simulink model "case 3"  (R2018a)
settings: Solver=VariableStepAuto  StartTime=0.0  StopTime=5  RelTol=1e-3
values from neighbouring files (symbols this model uses):
  cdcc = 0.00022    [matlab.mat]    (also in parameters.m)
  cf = 8e-05    [matlab.mat]    (also in parameters.m = 2e-05)
  iodmax = 12    [matlab.mat]    (also in parameters.m)
  iqdmax = -7.2    [matlab.mat]    (also in parameters.m)
  kiid = 0.5    [matlab.mat]    (also in parameters.m)
  kiiq = -5    [matlab.mat]    (also in parameters.m)
  kpid = 0.4    [matlab.mat]    (also in parameters.m)
  kpiq = -4    [matlab.mat]    (also in parameters.m)
  lf = 0.0075    [matlab.mat]    (also in parameters.m = 0.0015)
  ll = 1e-06    [matlab.mat]    (also in parameters.m)
  md = 0.001    [matlab.mat]    (also in parameters.m)
  nq = 0.002    [matlab.mat]    (also in parameters.m)
  p0 = 240    [matlab.mat]    (also in parameters.m)
  q0 = 60    [matlab.mat]    (also in parameters.m)
  rf = 0.0015    [matlab.mat]    (also in parameters.m)
  rl = 0.001    [matlab.mat]    (also in parameters.m)
  vdc = 200    [matlab.mat]    (also in parameters.m)
  wc = 0.000125663706144    [matlab.mat]    (also in parameters.m)
undefined symbols (not defined in the file or in its folder): DiscIntNeverNeededParam, gcbh, sps, sps_rtmsupport
libraries: powerlib_meascontrol x29, powerlib x17, simulink x6, spsVIMeasurementModel x6, spsMeanValueModel x2
(part 2 of 2)

== system case 3/Controller/Mean1/Mean1 ==
  In : Inport  SampleTime=Ts
  Model : Subsystem
  Mean : Outport  SampleTime=Ts
  wires:
  In/1 -> Model/1(In)
  Model/1(Mean) -> Mean/1

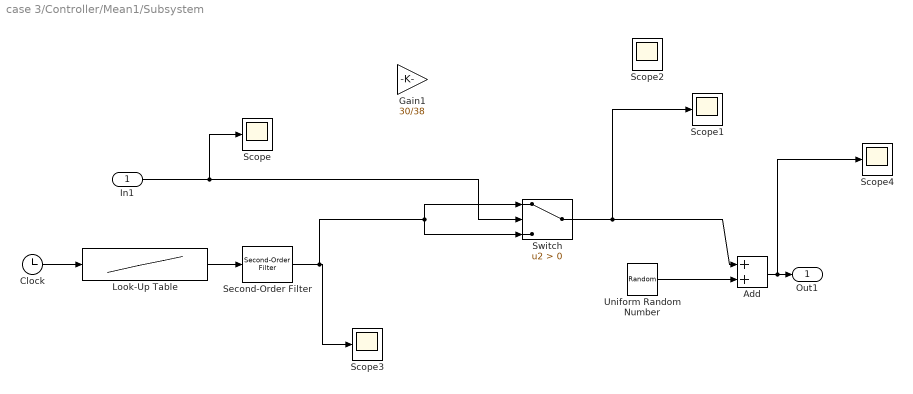
== system case 3/Controller/Mean1/Subsystem ==
  In1 : Inport
  Add : Sum
  Clock : Clock
  Gain1 : Gain  Gain=30/38
  Look-Up Table : Lookup  InputValues=[0 2 2.01 6]  Table=[-0.01 -0.01 -12 -12]  SaturateOnIntegerOverflow=on
  Scope{,1..4} (5 alike) : Scope
  Second-Order Filter : powerlib_meascontrol/Filters/Second-Order Filter  FilterType=Lowpass  Fo=10  Zeta=0.909  Ts=50e-6  Initialize=off  Vac_Init="[0,  0,  60]"  Vdc_Init=0  PlotResponse=off  FreqRange=[0, 500, 1]
      settings: SourceProductName=Simscape Power Systems  SourceProductBaseCode=PS
  Switch : Switch  Criteria=u2 > Threshold
  Uniform Random Number : UniformRandomNumber  Minimum=-0.5  Maximum=0.5  SampleTime=50e-6
  Out1 : Outport
  wires:
  Clock/1 -> Look-Up Table/1
  Look-Up Table/1 -> Second-Order Filter/1
  In1/1 -> Switch/2, Scope/1
  Second-Order Filter/1 -> Switch/1, Switch/3, Scope3/1
  Switch/1 -> Add/1, Scope1/1
  Add/1 -> Scope4/1, Out1/1
  Uniform Random Number/1 -> Add/2

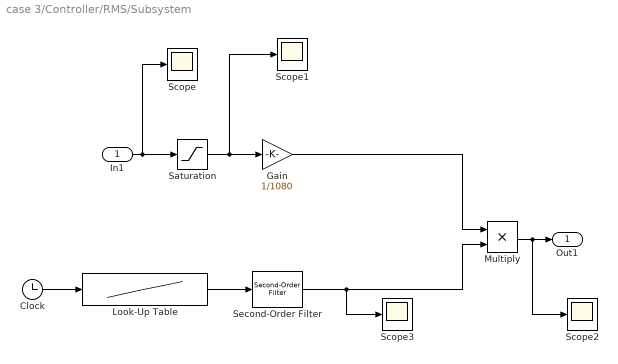
== system case 3/Controller/RMS/Subsystem ==
  In1 : Inport
  Clock : Clock
  Gain : Gain  Gain=1/1080
  Look-Up Table : Lookup  InputValues=[0 2 2.2 5]  Table=[235 235 80 120]  SaturateOnIntegerOverflow=on
  Multiply : Product
  Saturation : Saturate  UpperLimit=inf  LowerLimit=1080
  Scope{,1..3} (4 alike) : Scope
  Second-Order Filter : powerlib_meascontrol/Filters/Second-Order Filter  FilterType=Lowpass  Fo=30  Zeta=0.707  Ts=50e-6  Initialize=off  Vac_Init="[0,  0,  60]"  Vdc_Init=0  PlotResponse=off  FreqRange=[0, 500, 1]
      settings: SourceProductName=Simscape Power Systems  SourceProductBaseCode=PS
  Out1 : Outport
  wires:
  Saturation/1 -> Scope1/1, Gain/1
  In1/1 -> Scope/1, Saturation/1
  Gain/1 -> Multiply/1
  Clock/1 -> Look-Up Table/1
  Look-Up Table/1 -> Second-Order Filter/1
  Multiply/1 -> Scope2/1, Out1/1
  Second-Order Filter/1 -> Scope3/1, Multiply/2

== system case 3/Controller/RMS4/Mean1 ==
  In : Inport  SampleTime=Ts
  Model : Subsystem
  Mean : Outport  SampleTime=Ts
  wires:
  In/1 -> Model/1(In)
  Model/1(Mean) -> Mean/1

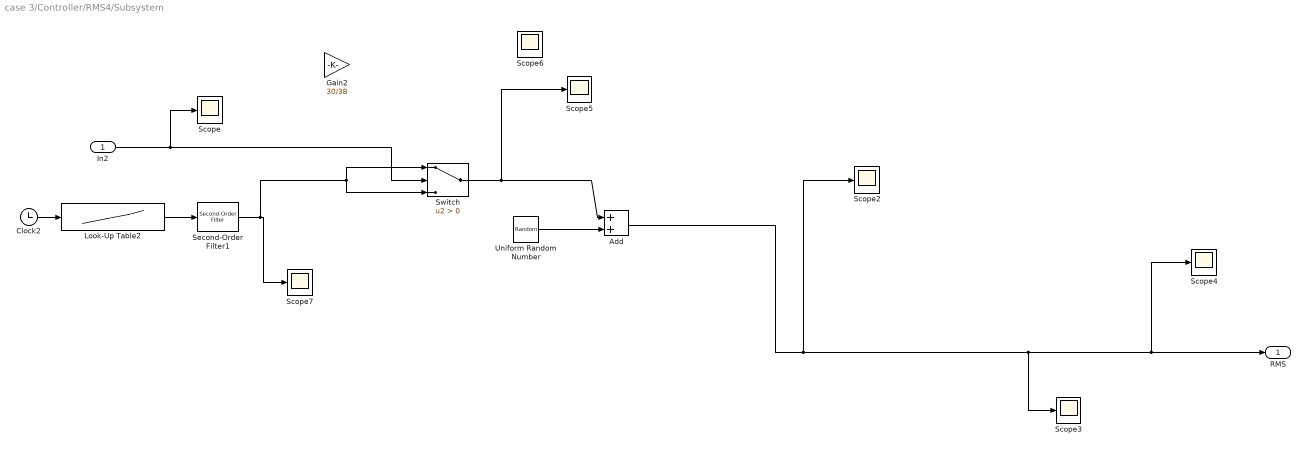
== system case 3/Controller/RMS4/Subsystem ==
  In2 : Inport
  Add : Sum
  Clock2 : Clock
  Gain2 : Gain  Gain=30/38
  Look-Up Table2 : Lookup  InputValues=[0 2 2.1 5]  Table=[50 50 480 480]  SaturateOnIntegerOverflow=on
  Scope{,2..7} (7 alike) : Scope
  Second-Order Filter1 : powerlib_meascontrol/Filters/Second-Order Filter  FilterType=Lowpass  Fo=50  Zeta=0.909  Ts=50e-6  Initialize=off  Vac_Init="[0,  0,  60]"  Vdc_Init=0  PlotResponse=off  FreqRange=[0, 500, 1]
      settings: SourceProductName=Simscape Power Systems  SourceProductBaseCode=PS
  Switch : Switch  Criteria=u2 > Threshold
  Uniform Random Number : UniformRandomNumber  SampleTime=50e-6
  RMS : Outport  SampleTime=Ts
  wires:
  Add/1 -> RMS/1, Scope4/1, Scope3/1, Scope2/1
  Uniform Random Number/1 -> Add/2
  Switch/1 -> Add/1, Scope5/1
  Second-Order Filter1/1 -> Switch/1, Switch/3, Scope7/1
  Look-Up Table2/1 -> Second-Order Filter1/1
  In2/1 -> Switch/2, Scope/1
  Clock2/1 -> Look-Up Table2/1

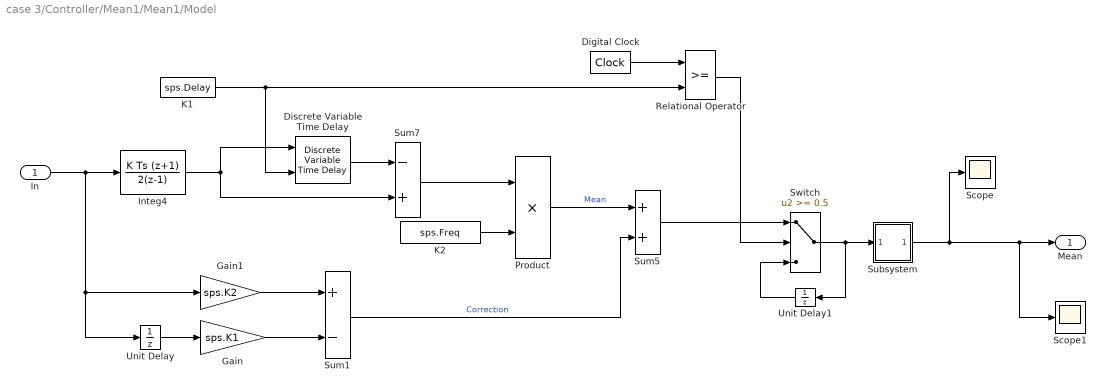
== system case 3/Controller/Mean1/Mean1/Model ==
  In : Inport
  Digital Clock : DigitalClock  SampleTime=Ts
  Discrete Variable Time Delay : powerlib_meascontrol/Additional Components/Discrete Variable Time Delay  MaxDelay=max(sps.Delay)+2*Ts  InitialValue=0  Ts=Ts  DFT=on
      settings: SourceProductName=Simscape Power Systems  SourceProductBaseCode=PS
  Gain : Gain  Gain=sps.K1  SaturateOnIntegerOverflow=on  OutDataTypeStr=Inherit: Same as input  ParamDataTypeStr=Inherit: Same as input
  Gain1 : Gain  Gain=sps.K2  SaturateOnIntegerOverflow=on  OutDataTypeStr=Inherit: Same as input  ParamDataTypeStr=Inherit: Same as input
  Integ4 : DiscreteIntegrator  IntegratorMethod=Integration: Trapezoidal  SampleTime=Ts  ICPrevOutput=DiscIntNeverNeededParam  ICPrevScaledInput=DiscIntNeverNeededParam
  K1 : Constant  Value=sps.Delay  SampleTime=Ts
  K2 : Constant  Value=sps.Freq  SampleTime=Ts
  Product : Product  SaturateOnIntegerOverflow=on  InputSameDT=on  OutDataTypeStr=Inherit: Same as first input
  Relational Operator : RelationalOperator  OutDataTypeStr=boolean  SampleTime=Ts  RndMeth=Nearest
  Scope : Scope
  Scope1 : Scope
  Subsystem : Subsystem
  Sum1 : Sum  Inputs=+-  SaturateOnIntegerOverflow=on  InputSameDT=on  OutDataTypeStr=Inherit: Same as first input
  Sum5 : Sum  SaturateOnIntegerOverflow=on  InputSameDT=on  OutDataTypeStr=Inherit: Same as first input
  Sum7 : Sum  Inputs=-+  SaturateOnIntegerOverflow=on  InputSameDT=on  OutDataTypeStr=Inherit: Same as first input
  Switch : Switch  Threshold=0.5  InputSameDT=on
  Unit Delay : UnitDelay  SampleTime=Ts
  Unit Delay1 : UnitDelay  InitialCondition=sps.Vinit  SampleTime=Ts
  Mean : Outport
  wires:
  Subsystem/1(Out1) -> Mean/1, Scope1/1, Scope/1
  Gain/1 -> Sum1/2
  Unit Delay/1 -> Gain/1
  Gain1/1 -> Sum1/1
  Discrete Variable Time Delay/1 -> Sum7/1
  Switch/1 -> Unit Delay1/1, Subsystem/1(In1)
  Sum5/1 -> Switch/1
  In/1 -> Unit Delay/1, Gain1/1, Integ4/1
  K2/1 -> Product/2
  Integ4/1 -> Sum7/2, Discrete Variable Time Delay/1
  Sum7/1 -> Product/1
  Product/1 -> Sum5/1  "Mean"
  Sum1/1 -> Sum5/2  "Correction"
  Unit Delay1/1 -> Switch/3
  Digital Clock/1 -> Relational Operator/1
  Relational Operator/1 -> Switch/2
  K1/1 -> Relational Operator/2, Discrete Variable Time Delay/2

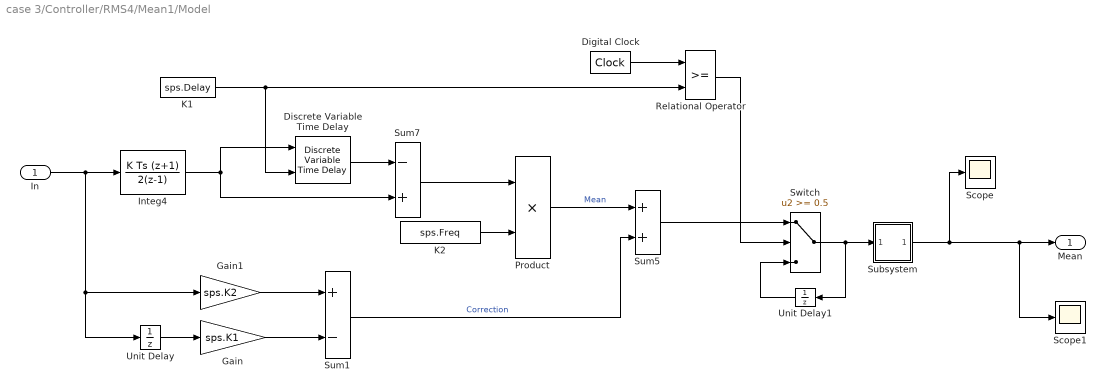
== system case 3/Controller/RMS4/Mean1/Model ==
  In : Inport
  Digital Clock : DigitalClock  SampleTime=Ts
  Discrete Variable Time Delay : powerlib_meascontrol/Additional Components/Discrete Variable Time Delay  MaxDelay=max(sps.Delay)+2*Ts  InitialValue=0  Ts=Ts  DFT=on
      settings: SourceProductName=Simscape Power Systems  SourceProductBaseCode=PS
  Gain : Gain  Gain=sps.K1  SaturateOnIntegerOverflow=on  OutDataTypeStr=Inherit: Same as input  ParamDataTypeStr=Inherit: Same as input
  Gain1 : Gain  Gain=sps.K2  SaturateOnIntegerOverflow=on  OutDataTypeStr=Inherit: Same as input  ParamDataTypeStr=Inherit: Same as input
  Integ4 : DiscreteIntegrator  IntegratorMethod=Integration: Trapezoidal  SampleTime=Ts  ICPrevOutput=DiscIntNeverNeededParam  ICPrevScaledInput=DiscIntNeverNeededParam
  K1 : Constant  Value=sps.Delay  SampleTime=Ts
  K2 : Constant  Value=sps.Freq  SampleTime=Ts
  Product : Product  SaturateOnIntegerOverflow=on  InputSameDT=on  OutDataTypeStr=Inherit: Same as first input
  Relational Operator : RelationalOperator  OutDataTypeStr=boolean  SampleTime=Ts  RndMeth=Nearest
  Scope : Scope
  Scope1 : Scope
  Subsystem : Subsystem
  Sum1 : Sum  Inputs=+-  SaturateOnIntegerOverflow=on  InputSameDT=on  OutDataTypeStr=Inherit: Same as first input
  Sum5 : Sum  SaturateOnIntegerOverflow=on  InputSameDT=on  OutDataTypeStr=Inherit: Same as first input
  Sum7 : Sum  Inputs=-+  SaturateOnIntegerOverflow=on  InputSameDT=on  OutDataTypeStr=Inherit: Same as first input
  Switch : Switch  Threshold=0.5  InputSameDT=on
  Unit Delay : UnitDelay  SampleTime=Ts
  Unit Delay1 : UnitDelay  InitialCondition=sps.Vinit  SampleTime=Ts
  Mean : Outport
  wires:
  Subsystem/1(Out1) -> Mean/1, Scope1/1, Scope/1
  Gain/1 -> Sum1/2
  Unit Delay/1 -> Gain/1
  Gain1/1 -> Sum1/1
  Discrete Variable Time Delay/1 -> Sum7/1
  Switch/1 -> Unit Delay1/1, Subsystem/1(In1)
  Sum5/1 -> Switch/1
  In/1 -> Unit Delay/1, Gain1/1, Integ4/1
  K2/1 -> Product/2
  Integ4/1 -> Sum7/2, Discrete Variable Time Delay/1
  Sum7/1 -> Product/1
  Product/1 -> Sum5/1  "Mean"
  Sum1/1 -> Sum5/2  "Correction"
  Unit Delay1/1 -> Switch/3
  Digital Clock/1 -> Relational Operator/1
  Relational Operator/1 -> Switch/2
  K1/1 -> Relational Operator/2, Discrete Variable Time Delay/2

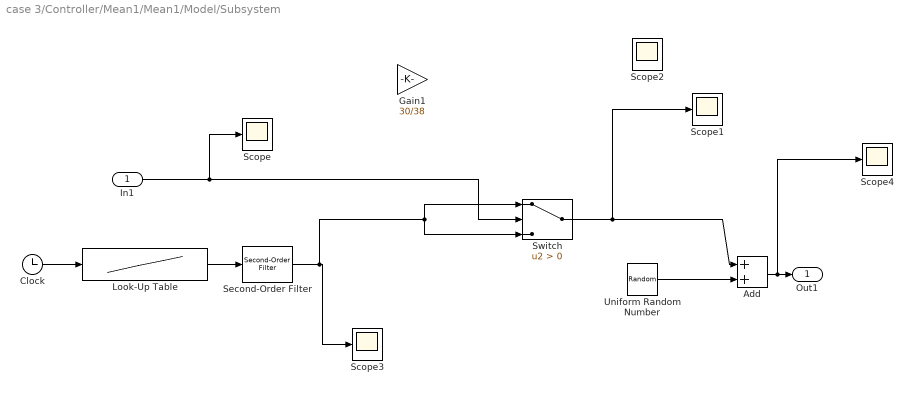
== system case 3/Controller/Mean1/Mean1/Model/Subsystem ==
  In1 : Inport
  Add : Sum
  Clock : Clock
  Gain1 : Gain  Gain=30/38
  Look-Up Table : Lookup  InputValues=[0 2 2.01 6]  Table=[-0.01 -0.01 -8 -8]  SaturateOnIntegerOverflow=on
  Scope{,1..4} (5 alike) : Scope
  Second-Order Filter : powerlib_meascontrol/Filters/Second-Order Filter  FilterType=Lowpass  Fo=10  Zeta=0.909  Ts=50e-6  Initialize=off  Vac_Init="[0,  0,  60]"  Vdc_Init=0  PlotResponse=off  FreqRange=[0, 500, 1]
      settings: SourceProductName=Simscape Power Systems  SourceProductBaseCode=PS
  Switch : Switch  Criteria=u2 > Threshold
  Uniform Random Number : UniformRandomNumber  Minimum=-0.7  Maximum=0.7  SampleTime=50e-6
  Out1 : Outport
  wires:
  Clock/1 -> Look-Up Table/1
  Look-Up Table/1 -> Second-Order Filter/1
  In1/1 -> Switch/2, Scope/1
  Second-Order Filter/1 -> Switch/1, Switch/3, Scope3/1
  Switch/1 -> Add/1, Scope1/1
  Add/1 -> Scope4/1, Out1/1
  Uniform Random Number/1 -> Add/2

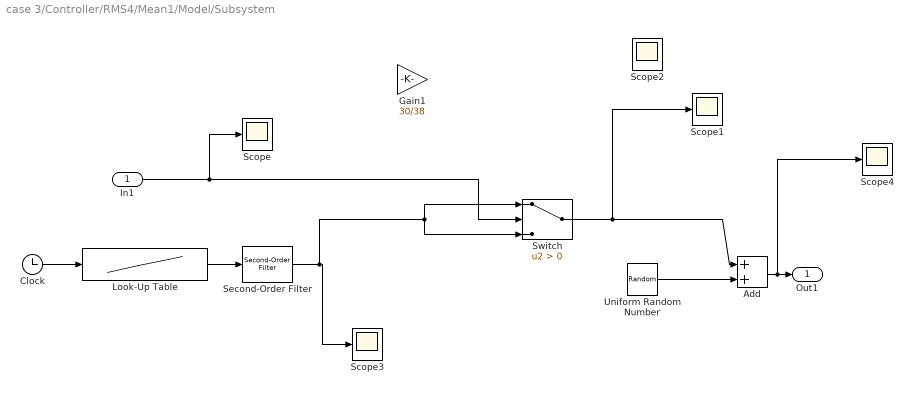
== system case 3/Controller/RMS4/Mean1/Model/Subsystem ==
  In1 : Inport
  Add : Sum
  Clock : Clock
  Gain1 : Gain  Gain=30/38
  Look-Up Table : Lookup  InputValues=[0 2 2.01 6]  Table=[-0.01 -0.01 -8 -8]  SaturateOnIntegerOverflow=on
  Scope{,1..4} (5 alike) : Scope
  Second-Order Filter : powerlib_meascontrol/Filters/Second-Order Filter  FilterType=Lowpass  Fo=10  Zeta=0.909  Ts=50e-6  Initialize=off  Vac_Init="[0,  0,  60]"  Vdc_Init=0  PlotResponse=off  FreqRange=[0, 500, 1]
      settings: SourceProductName=Simscape Power Systems  SourceProductBaseCode=PS
  Switch : Switch  Criteria=u2 > Threshold
  Uniform Random Number : UniformRandomNumber  Minimum=-0.1  Maximum=0.1  SampleTime=50e-6
  Out1 : Outport
  wires:
  Clock/1 -> Look-Up Table/1
  Look-Up Table/1 -> Second-Order Filter/1
  In1/1 -> Switch/2, Scope/1
  Second-Order Filter/1 -> Switch/1, Switch/3, Scope3/1
  Switch/1 -> Add/1, Scope1/1
  Add/1 -> Scope4/1, Out1/1
  Uniform Random Number/1 -> Add/2
